simulink model "b2b_th2"  (R2018a)
settings: Solver=VariableStepAuto  StartTime=0.0  StopTime=50  RelTol=1e-3
libraries: simulink x2
settings Model: Creator=Huy  LastModifiedBy=Huy

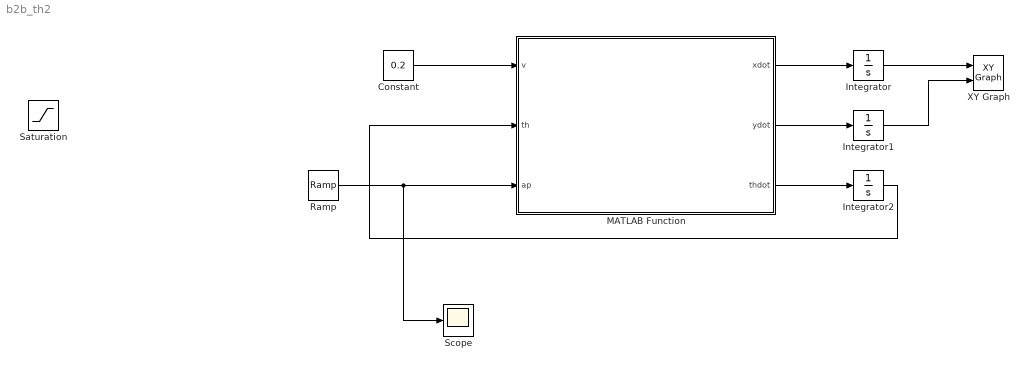
== system b2b_th2 ==
  Constant : Constant  Value=0.2
  Integrator : Integrator
  Integrator1 : Integrator
  Integrator2 : Integrator
  MATLAB Function : MATLAB Function  TreatAsAtomicUnit=on
  Ramp : simulink/Sources/Ramp  slope=1  start=0  InitialOutput=0
  Saturation : Saturate
  Scope : Scope
  XY Graph : simulink/Sinks/XY Graph  xmin=-1  xmax=5  ymin=-1  ymax=5  st=1
  wires:
  MATLAB Function/1(xdot) -> Integrator/1
  Constant/1 -> MATLAB Function/1(v)
  MATLAB Function/2(ydot) -> Integrator1/1
  MATLAB Function/3(thdot) -> Integrator2/1
  Integrator/1 -> XY Graph/1
  Integrator1/1 -> XY Graph/2
  Integrator2/1 -> MATLAB Function/2(th)
  Ramp/1 -> Scope/1, MATLAB Function/3(ap)

== matlab function b2b_th2/MATLAB Function ==
  data: v input; xdot output; th input; ap input; ydot output; thdot output
function [xdot,ydot,thdot] = tricycle (v,th,ap)
vmax = 0.36; 
amax = 0.28;
apmax = (pi/4)*180/pi 
wmax = 0.30;  
G = 13;
d = sqrt(2.5 + 0.1*G);
xdot = v*cos(th);
ydot = v*sin(th);
thdot = v/d *sin(ap);
%vc = v/cos(alpha);
%vcmax=0.36/sqrt(2)/2=0.509m/s;                                
%vcmin = 0 m/s;
